simulink model "full_maneuver_platoon_new_strategy"  (R2019a)
settings: Solver=VariableStepAuto  StartTime=0.0  StopTime=70  FixedStep=0.1  MaxStep=0.05  RelTol=1e-3
libraries: simulink x97, dspsigops x7, powerlib_meascontrol x7, autolibshared x7
(part 7 of 7)

== stateflow chart full_maneuver_platoon_new_strategy/p1/Virtual Vehicle Following/Chart ==
  state VehFollowing
    during:
    u = uVehFoll;
    state = 0;
  state SpeedControl
    during:
    u = uVelControl;
    state = 1;
  (default) -> VehFollowing
  SpeedControl -> VehFollowing : [uVehFoll>=uVelControl]
  VehFollowing -> SpeedControl : [(velDiff>=0) && (uVehFoll<0)]
  data: state output size=1; u output size=1; velDiff input size=1; uVelControl input double; uVehFoll input size=1

== stateflow chart full_maneuver_platoon_new_strategy/p2/Regular Vehicle Following/Chart ==
  state VehFollowing
    during:
    u = vehFoll;
    state = 0;
  state FreeFlowVelControl
    during:
    u = freeFlowVelControl;
    state = 1;
  state MinVelControl
    during:
    u = minVelControl;
    state = 1;
  (default) -> VehFollowing
  VehFollowing -> MinVelControl [order 1] : [(velDiff>=0) && (vehFoll<0) && (~unsafeFlag)]
  VehFollowing -> FreeFlowVelControl [order 2] : [leaderWithinRange==0]
  FreeFlowVelControl -> VehFollowing : [leaderWithinRange==1]
  MinVelControl -> VehFollowing : [(vehFoll>=minVelControl) || unsafeFlag]
  data: state output size=1; u output size=1; leaderWithinRange input size=1; velDiff input; unsafeFlag input; vehFoll input size=1; freeFlowVelControl input double; minVelControl input

== stateflow chart full_maneuver_platoon_new_strategy/p2/Vehicle Following During LC/Chart ==
  state VehFollowing
    during:
    u = uVehFoll;
    state = 0;
  state SpeedControl
    during:
    u = uVelControl;
    state = 1;
  (default) -> VehFollowing
  SpeedControl -> VehFollowing : [leaderWithinRange==1]
  VehFollowing -> SpeedControl : [leaderWithinRange==0]
  data: state output size=1; u output size=1; leaderWithinRange input size=1; uVehFoll input size=1; uVelControl input double

== stateflow chart full_maneuver_platoon_new_strategy/p2/Virtual Vehicle Following/Chart ==
  state VehFollowing
    during:
    u = uVehFoll;
    state = 0;
  state SpeedControl
    during:
    u = uVelControl;
    state = 1;
  (default) -> VehFollowing
  SpeedControl -> VehFollowing : [uVehFoll>=uVelControl]
  VehFollowing -> SpeedControl : [(velDiff>=0) && (uVehFoll<0)]
  data: state output size=1; u output size=1; velDiff input size=1; uVelControl input double; uVehFoll input size=1

== stateflow chart full_maneuver_platoon_new_strategy/p3/ControlChoice ==
  state RegVehFoll
    entry:
    state = 1;
    during:
    data = regVehFollData;
  state AdjForLaneChange
    entry:
    state = 2;
    during:
    if leaderInRange
    data = min(regVehFollData, longAdjustmentData);
    else
    data = longAdjustmentData;
    end
  state LaneChanging
    entry:
    state = 3;
    during:
    if leaderInRange
    data = min(regVehFollData, laneChangingData);
    else
    data = laneChangingData;
    end
  (default) -> RegVehFoll
  LaneChanging -> RegVehFoll : [laneChangeDone]
  RegVehFoll -> LaneChanging [order 2] : [laneChangeStarted && ~laneChangeDone]
  RegVehFoll -> AdjForLaneChange [order 1] : [startAdjustment && ~laneChangeStarted]
  AdjForLaneChange -> LaneChanging : [laneChangeStarted]
  data: regVehFollData input; longAdjustmentData input; laneChangingData input; startAdjustment input size=1; data output; laneChangeStarted input; state output; laneChangeDone input; leaderInRange input

== matlab function full_maneuver_platoon_new_strategy/p3/MATLAB Function ==
  data: leader output Bus: vehStatesBus; ego input Bus: vehStatesBus; allVehicles input; indices output; lcFlag input
function [leader, indices] = findLeader(ego, allVehicles, lcFlag)

nv = length(allVehicles);

leaderIdx = -1;

farAwayVehicle.X = ego.X + 10^4;
farAwayVehicle.Y = ego.Y;
farAwayVehicle.Xdot = ego.Xdot;
farAwayVehicle.u = 0;

leader = farAwayVehicle;

% For non lane changing vehicles, the leader is whoever is longitudinally
% closer and with any part of the body in the same lane
if ~lcFlag
    for n = 1:nv
        if allVehicles(n).X>ego.X && allVehicles(n).X<leader.X
            if abs(allVehicles(n).Y - ego.Y)<=2.7 % 1.8 (half lane) + 0.9 (half veh width)
                leader = allVehicles(n);
                leaderIdx=n;
            end
        end
    end
% For lane changing vehicles, we want to keep the original leader until the
% ego vehicle is out of the lane
else
    for n = 1:nv
        if allVehicles(n).X>ego.X && allVehicles(n).X<leader.X
            if abs(allVehicles(n).Y - ego.Y)<=1.9 % 1.8 (half lane) + 0.9 (half veh width)
                leader = allVehicles(n);
                leaderIdx=n;
            end
        end
    end
end

indices = leaderIdx;

== stateflow chart full_maneuver_platoon_new_strategy/p3/Regular Vehicle Following/Chart ==
  state VehFollowing
    during:
    u = vehFoll;
    state = 0;
  state FreeFlowVelControl
    during:
    u = freeFlowVelControl;
    state = 1;
  state MinVelControl
    during:
    u = minVelControl;
    state = 1;
  (default) -> VehFollowing
  VehFollowing -> MinVelControl [order 1] : [(velDiff>=0) && (vehFoll<0) && (~unsafeFlag)]
  VehFollowing -> FreeFlowVelControl [order 2] : [leaderWithinRange==0]
  FreeFlowVelControl -> VehFollowing : [leaderWithinRange==1]
  MinVelControl -> VehFollowing : [(vehFoll>=minVelControl) || unsafeFlag]
  data: state output size=1; u output size=1; leaderWithinRange input size=1; velDiff input; unsafeFlag input; vehFoll input size=1; freeFlowVelControl input double; minVelControl input

== stateflow chart full_maneuver_platoon_new_strategy/p3/Vehicle Following During LC/Chart ==
  state VehFollowing
    during:
    u = uVehFoll;
    state = 0;
  state SpeedControl
    during:
    u = uVelControl;
    state = 1;
  (default) -> VehFollowing
  SpeedControl -> VehFollowing : [leaderWithinRange==1]
  VehFollowing -> SpeedControl : [leaderWithinRange==0]
  data: state output size=1; u output size=1; leaderWithinRange input size=1; uVehFoll input size=1; uVelControl input double

== stateflow chart full_maneuver_platoon_new_strategy/p3/Virtual Vehicle Following/Chart ==
  state VehFollowing
    during:
    u = uVehFoll;
    state = 0;
  state SpeedControl
    during:
    u = uVelControl;
    state = 1;
  (default) -> VehFollowing
  SpeedControl -> VehFollowing : [uVehFoll>=uVelControl]
  VehFollowing -> SpeedControl : [(velDiff>=0) && (uVehFoll<0)]
  data: state output size=1; u output size=1; velDiff input size=1; uVelControl input double; uVehFoll input size=1
